simulink model "automotive_console_test"  (R2020b)
settings: Solver=VariableStepAuto  StartTime=0.0  StopTime=10.0  RelTol=1e-3
undefined symbols (not defined in the file): sigbuilder_block
settings Model: Creator=Milind  LastModifiedBy=Milind

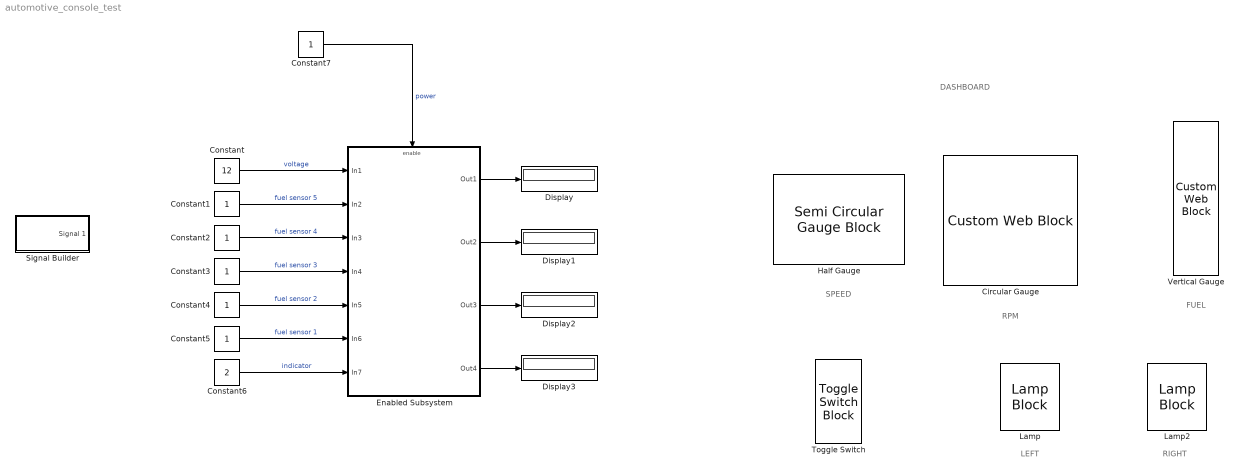
== system automotive_console_test ==
  note: LEFT
  note: SPEED
  note: DASHBOARD
  note: RIGHT
  note: RPM
  note: FUEL
  Circular Gauge : CustomWebBlock  LabelPosition=Hide  ShowInitialText=on  Configuration="{\"components\":[{\"name\":\"CircularScaleComponent\",\"settings\":{\"bounds\":{\"max\":10,\"min\":0,\"tickInterval\":\"auto\"},\"direction\":\"cw\",\"flipLimits\":0,\"innerRadius\":0.75,\"internalTickHeightScaleFactor\":1,\"labelColor\":[255,252,199],\"labelFont\":{\"font\":\"Arial\",\"fontSize\":12},\"labelTransparency\":1,\"minorTickHeightScaleFactor\":0.2,\"needleImage\":{\"size\":[1890,567],\"src\":\"data:image\\/svg+xml;base64,PD94bWwgdmVyc2lvbj0iMS4wIiBlbmNvZGluZz0iVVRGLTgiIHN0YW5kYWxvbmU9Im5vIj8+CjxzdmcKICAgeG1sbnM6ZGM9Imh0dHA6Ly9wdXJsLm9yZy9kYy9lbGVtZW50cy8xLjEvIgogICB4bWxuczpjYz0iaHR0cDovL2NyZWF0aXZlY29tbW9ucy5vcmcvbnMjIgogICB4bWxuczpyZGY9Imh0dHA6Ly93d3cudzMub3JnLzE5OTkvMDIvMjItcmRmLXN5bnRheC1ucyMiCiAgIHhtbG5zOnN2Zz0iaHR0cDovL3d3dy53My5vcmcvMjAwMC9zdmciCiAgIHhtbG5zPSJodHRwOi8vd3d3LnczLm9yZy8yMDAwL3N2ZyIKICAgeG1sbnM6 ...(+4096 chars)\"},\"needleOffset\":[0.1610917094974375,0],\"needleOrientation\":-45,\"needleRotation\":180.59702388394928,\"needleSize\":{\"height\":0.13032601008944536,\"width\":0.416859542883425},\"outerRadius\":0.9,\"position\":[0.06486742424242424,0.05627705627705628,0.8917748917748918,0.8787878787878788],\"scaleAngle\":270,\"scaleAngleOffset\":135,\"scaleColors\":[],\"scaleColorsSize\":0.2,\"scalePosition\":[0,0,1,1],\"showLabels\":1,\"showMinorTicks\":1,\"showSpanLine\":1,\"showTicks\":1,\"tickColor\":[255,255,200],\"tickTransparency\":1,\"valueBarColor\":[0,114,189],\"valueBarPosition\":[0,0,1,1],\"valueBarSize\":0.2,\"valueBarTransparency\":1}},{\"name\":\"BackgroundImageComponent\",\"settings\":{\"image\":{\"size\":[500,500],\"src\":\"data:image\\/svg+xml;base64,PD94bWwgdmVyc2lvbj0iMS4wIiBlbmNvZGluZz0iVVRGLTgiIHN0YW5kYWxvbmU9Im5vIj8+CjxzdmcKICAgeG1sbnM6ZGM9Imh0dHA6Ly9wdXJsLm9yZy9kYy9lbGVtZW50cy8xLjEvIgogICB4bWxuczpjYz0iaHR0cDovL2NyZWF0aXZlY29tbW9ucy5vcmcvbnMjIgogICB4bWxuczpyZGY9Imh0dHA6Ly93d3cudzMub3JnLzE5OTkvMDIvMjItcmRmLXN5bnRheC1ucyMiCiAgIHhtbG5zOnN2Zz0iaHR0cDovL3d3dy53My5vcmcvMjAwMC9zdmciCiAgIHhtbG5zPSJodHRwOi8vd3d3LnczLm9yZy8yMDAwL3N2ZyIKICAgeG1sbnM6 ...(+9964 chars)\"},\"position\":[0,0,1,1],\"scaleMode\":\"0\"}},{\"name\":\"ForegroundImageComponent\",\"settings\":{\"image\":{\"size\":[0,0],\"src\":\"default\",\"srcOrientation\":[]},\"isForeground\":1,\"position\":[0,0,1,1],\"scaleMode\":\"0\"}}],\"settings\":{\"BindingType\":\"signal\",\"aspectRatio\":1.032258064516129,\"direction\":\"cw\",\"fixedAspectRatio\":\"on\",\"flipLimits\":0,\"orientation\":\"horizontal\"},\"type\":\"CircularGauge\"}"
  Constant : Constant  Value=12
  Constant{1..5,7} (6 alike) : Constant
  Constant6 : Constant  Value=2
  Display{,1..3} (4 alike) : Display
  Enabled Subsystem : Subsystem  TreatAsAtomicUnit=on
  Half Gauge : SemiCircularGaugeBlock
  Lamp : LampBlock
  Lamp2 : LampBlock
  Signal Builder : Subsystem  Tag=STV Subsys  LoadFcn=sigbuilder_block('load');  StartFcn=sigbuilder_block('start');  StopFcn=sigbuilder_block('stop');  ClipboardFcn=sigbuilder_block('clipboard');  mask(Sigbuilder block){tuvar=[0:10]}
      mask help: Simulink:masks:SigbuilderBlock_MD
      mask init:
      | if ~strcmp(get_param(bdroot(gcbh),'SimulationStatus'),'stopped') tuvar = sigbuilder_block('maskInit'); end
      settings: CopyFcn=sigbuilder_block('copy');  DeleteFcn=sigbuilder_block('delete');  ModelCloseFcn=sigbuilder_block('modelClose');  PreSaveFcn=sigbuilder_block('preSave');  PauseFcn=sigbuilder_block('pause');  ContinueFcn=sigbuilder_block('continue');  NameChangeFcn=sigbuilder_block('namechange');  OpenFcn=sigbuilder_block('open',[437.6 153 550.4 359.25 ]);  CloseFcn=sigbuilder_block('close');
      mask Display: plot(0, 0, 100, 100,[2, 2, 32, 32, 2], [68, 8, 8, 68, 68],[32, 2], [38, 38], [32, 19, 2],[53, 60, 44], [32, 17, 17, 2],[16, 16, 31, 31]);txt = getActiveGroup(gcbh);text(2, 100, txt,'verticalAlignment', 'top');
  Toggle Switch : ToggleSwitchBlock
      settings: Values={{'Off', 'On'}, [0 1]}
  Vertical Gauge : CustomWebBlock  ShowInitialText=on  Configuration="{\"components\":[{\"name\":\"LinearScaleComponent\",\"settings\":{\"bounds\":{\"max\":5,\"min\":0,\"tickInterval\":\"auto\"},\"internalTickHeightScaleFactor\":0.5,\"labelColor\":[250,245,199],\"labelFont\":{\"font\":\"Arial\",\"fontSize\":12},\"labelTransparency\":1,\"needleImage\":{\"size\":[21,75],\"src\":\"data:image\\/svg+xml;base64,PHN2ZyB4bWxucz0iaHR0cDovL3d3dy53My5vcmcvMjAwMC9zdmciIHhtbG5zOnhsaW5rPSJodHRwOi8vd3d3LnczLm9yZy8xOTk5L3hsaW5rIiB2aWV3Qm94PSIwIDAgMjEgNzUiPjxkZWZzPjxzdHlsZT4uY2xzLTF7ZmlsbDpub25lO30uY2xzLTJ7aXNvbGF0aW9uOmlzb2xhdGU7fS5jbHMtM3tjbGlwLXBhdGg6dXJsKCNjbGlwLXBhdGgpO30uY2xzLTR7b3BhY2l0eTowLjM7bWl4LWJsZW5kLW1vZGU6bXVsdGlwbHk7fS5jbHMtNXtmaWxsOiNlYjI2Mjk7fTwvc3R5bGU+PGNsaXBQYXRoIGlkPSJjbGlwLXBhdGgiIHRyYW5zZm9y ...(+1928 chars)\",\"srcOrientation\":\"horizontal\"},\"needleOffset\":[-0.01094391244870041,0],\"needleSize\":{\"height\":0.11960078534031414,\"width\":0.7589285714285714},\"position\":[0.015887605042016806,0.06986607142857143,0.8,0.9641544117647058],\"scaleColors\":[],\"scaleColorsSize\":0.2,\"showLabels\":1,\"showMinorTicks\":0,\"showSpanLine\":1,\"showTicks\":1,\"tickColor\":[250,245,200],\"tickTransparency\":1,\"valueBarColor\":[23,89,176],\"valueBarOffset\":0,\"valueBarSize\":0.23,\"valueBarTransparency\":1}},{\"name\":\"BackgroundImageComponent\",\"settings\":{\"image\":{\"size\":[101,380],\"src\":\"data:image\\/svg+xml;base64,PHN2ZyB4bWxucz0iaHR0cDovL3d3dy53My5vcmcvMjAwMC9zdmciIHZpZXdCb3g9IjAgMCAxMDEgMzgwIj48ZGVmcz48c3R5bGU+LmNscy0xe2ZpbGw6IzAwMmI0Mjt9LmNscy0ye2ZpbGw6IzQyNzA4Mjt9LmNscy0ze2ZpbGw6IzdjYTBiMjt9PC9zdHlsZT48L2RlZnM+PHRpdGxlPnZlcnRpY2FsX2dhdWdlX2JhY2tncm91bmRfMTwvdGl0bGU+PGcgaWQ9IkxheWVyXzIiIGRhdGEtbmFtZT0iTGF5ZXIgMiI+PGcgaWQ9IkxheWVyXzEtMiIgZGF0YS1uYW1lPSJMYXllciAxIj48cmVjdCBjbGFzcz0iY2xzLTEiIHg9IjExIiB5PSIxMSIgd2lkdGg9Ijc5IiBoZWlnaHQ9IjM1OCIvPjxwYXRoIGNsYXNzPSJjbHMtMiIgZD0iTTkzLDhIOFYzNzJIOTNaTTExLDM2OVYxMUg5MFYzNjlaIi8+PHBhdGggY2xhc3M9ImNscy0zIiBkPSJNMTAxLDBIMFYzODBIMTAxWk04LDM3MlY4SDkzVjM3MloiLz48L2c+PC9nPjwvc3ZnPg==\",\"srcOrientation\":\"vertical\"},\"position\":[0,0,1,1],\"scaleMode\":\"0\"}},{\"name\":\"ForegroundImageComponent\",\"settings\":{\"image\":{\"size\":[0,0],\"src\":\"default\",\"srcOrientation\":[]},\"isForeground\":1,\"position\":[0,0,1,1],\"scaleMode\":\"0\"}}],\"settings\":{\"BindingType\":\"signal\",\"aspectRatio\":0.2647058823529412,\"fixedAspectRatio\":\"on\",\"orientation\":\"vertical\"},\"type\":\"LinearGauge\"}"
  wires:
  Enabled Subsystem/2(Out2) -> Display1/1
  Enabled Subsystem/3(Out3) -> Display2/1
  Constant2/1 -> Enabled Subsystem/3(In3)  "fuel sensor 4"
  Enabled Subsystem/1(Out1) -> Display/1
  Enabled Subsystem/4(Out4) -> Display3/1
  Constant7/1 -> Enabled Subsystem/Enable  "power"
  Constant5/1 -> Enabled Subsystem/6(In6)  "fuel sensor 1"
  Constant3/1 -> Enabled Subsystem/4(In4)  "fuel sensor 3"
  Constant6/1 -> Enabled Subsystem/7(In7)  "indicator"
  Constant4/1 -> Enabled Subsystem/5(In5)  "fuel sensor 2"
  Constant/1 -> Enabled Subsystem/1(In1)  "voltage"
  Constant1/1 -> Enabled Subsystem/2(In2)  "fuel sensor 5"

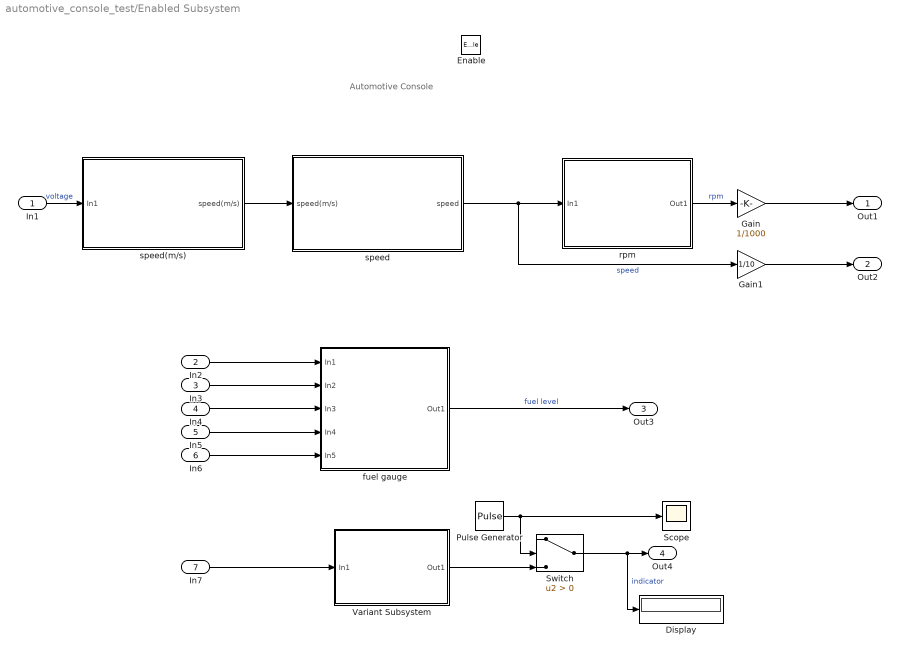
== system automotive_console_test/Enabled Subsystem ==
  note: Automotive Console
  In1 : Inport
  In2 : Inport  Port=2
  In3 : Inport  Port=3
  In4 : Inport  Port=4
  In5 : Inport  Port=5
  In6 : Inport  Port=6
  In7 : Inport  Port=7
  Enable : EnablePort
  Display : Display
  Gain : Gain  Gain=1/1000
  Gain1 : Gain  Gain=1/10
  Pulse Generator : DiscretePulseGenerator  PulseType=Time based  PulseWidth=50
  Scope : Scope
  Switch : Switch  Criteria=u2 > Threshold
  Variant Subsystem : Subsystem  Variant=on
  fuel gauge : Subsystem
  rpm : Subsystem  Variant=on
  speed : Subsystem  Variant=on  AllowZeroVariantControls=on
  speed(m/s) : Subsystem
  Out1 : Outport
  Out2 : Outport  Port=2
  Out3 : Outport  Port=3
  Out4 : Outport  Port=4
  wires:
  fuel gauge/1(Out1) -> Out3/1  "fuel level"
  Variant Subsystem/1(Out1) -> Switch/3
  speed/1(speed) -> Gain1/1, rpm/1(In1)  "speed"
  In2/1 -> fuel gauge/1(In1)
  In3/1 -> fuel gauge/2(In2)
  In4/1 -> fuel gauge/3(In3)
  rpm/1(Out1) -> Gain/1  "rpm"
  Pulse Generator/1 -> Scope/1, Switch/2
  In5/1 -> fuel gauge/4(In4)
  In7/1 -> Variant Subsystem/1(In1)
  In1/1 -> speed(m/s)/1(In1)  "voltage"
  In6/1 -> fuel gauge/5(In5)
  speed(m/s)/1(speed(m/s)) -> speed/1(speed(m/s))
  Switch/1 -> Display/1, Out4/1  "indicator"
  Gain/1 -> Out1/1
  Gain1/1 -> Out2/1

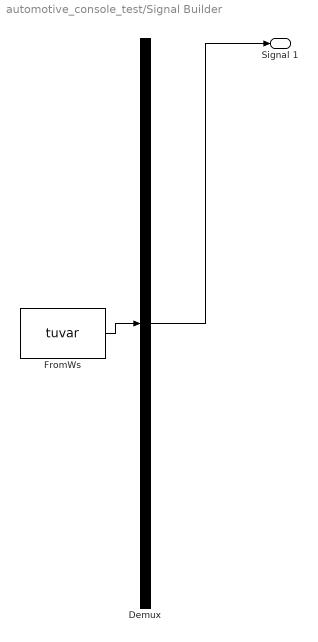
== system automotive_console_test/Signal Builder ==
  Demux : Demux  Tag=STV Demux  Outputs=1
      settings: DisplayOption=none
  FromWs : FromWorkspace  Tag=STV FromWs  VariableName=tuvar
      SigBuilderData=|
      | common.afterFinalStr = 'Extrapolate'
      | common.sampleTime = 0
      | dataSet.timeRange = [0 10]
      | dataSet.name = 'Group 1'
      | sbobj.Groups.Name = 'Group 1'
      | sbobj.Groups.Signals.Name = 'Signal 1'
      | sbobj.Groups.Signals.XData = [0 4 4 6 6 10]
      | sbobj.Groups.Signals.YData = [0 0 1 1 0 0]
  Signal 1 : Outport  Tag=STV Outport
  wires:
  Demux/1 -> Signal 1/1
  FromWs/1 -> Demux/1

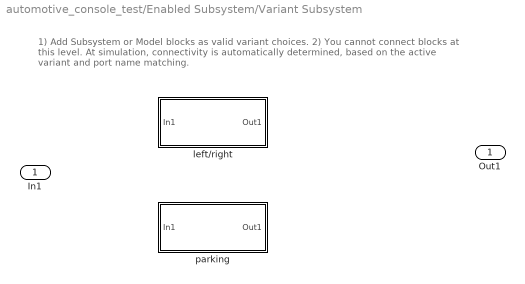
== system automotive_console_test/Enabled Subsystem/Variant Subsystem ==
  note: 1) Add Subsystem or Model blocks as valid variant choices.
      | 2) You cannot connect blocks at this level. At simulation, connectivity is automatically
      | determined, based on the active variant and port name matching.
  In1 : Inport
  left/right : Subsystem  VariantControl=ind==0
  parking : Subsystem  VariantControl=ind==1
  Out1 : Outport

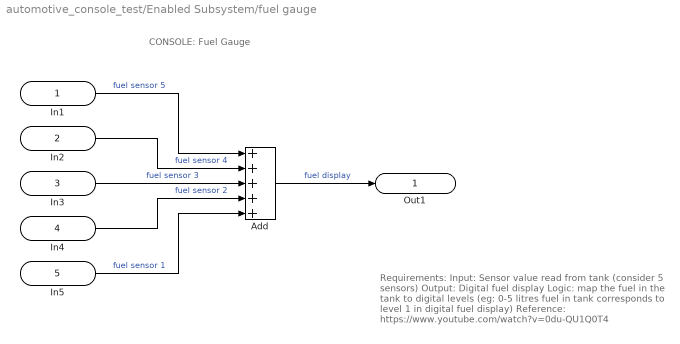
== system automotive_console_test/Enabled Subsystem/fuel gauge ==
  note: CONSOLE: Fuel Gauge
  note: Requirements:
      | Input: Sensor value read from tank (consider 5 sensors)
      | Output: Digital fuel display
      | Logic: map the fuel in the tank to digital levels (eg: 0-5 litres fuel in tank corresponds to level 1 in digital fuel display) Reference: https://www.youtube.com/watch?v=0du-QU1Q0T4
  In1 : Inport
  In2 : Inport  Port=2
  In3 : Inport  Port=3
  In4 : Inport  Port=4
  In5 : Inport  Port=5
  Add : Sum  Inputs=+++++
  Out1 : Outport
  wires:
  Add/1 -> Out1/1  "fuel display"
  In1/1 -> Add/1  "fuel sensor 5"
  In2/1 -> Add/2  "fuel sensor 4"
  In3/1 -> Add/3  "fuel sensor 3"
  In4/1 -> Add/4  "fuel sensor 2"
  In5/1 -> Add/5  "fuel sensor 1"

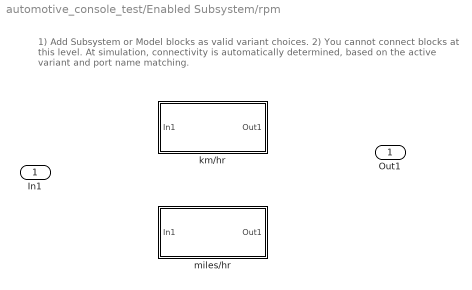
== system automotive_console_test/Enabled Subsystem/rpm ==
  note: 1) Add Subsystem or Model blocks as valid variant choices.
      | 2) You cannot connect blocks at this level. At simulation, connectivity is automatically
      | determined, based on the active variant and port name matching.
  In1 : Inport
  km/hr : Subsystem  VariantControl=control==0
  miles/hr : Subsystem  VariantControl=control==1
  Out1 : Outport

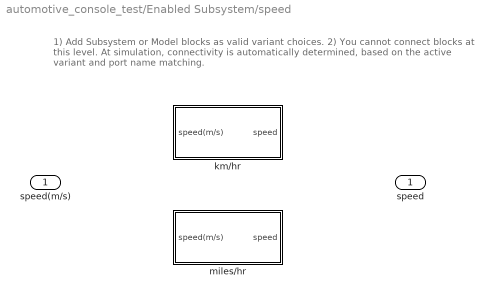
== system automotive_console_test/Enabled Subsystem/speed ==
  note: 1) Add Subsystem or Model blocks as valid variant choices.
      | 2) You cannot connect blocks at this level. At simulation, connectivity is automatically
      | determined, based on the active variant and port name matching.
  speed(m/s) : Inport
  km/hr : Subsystem  VariantControl=control==0
  miles/hr : Subsystem  VariantControl=control==1
  speed : Outport

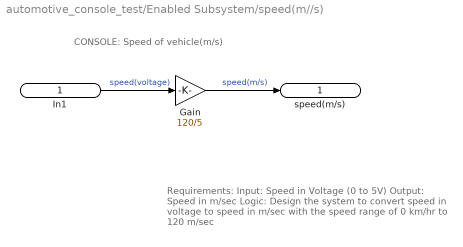
== system automotive_console_test/Enabled Subsystem/speed(m//s) ==
  note: CONSOLE: Speed of vehicle(m/s)
  note: Requirements:
      | Input: Speed in Voltage (0 to 5V)
      | Output: Speed in m/sec
      | Logic: Design the system to convert speed in voltage to
      | speed in m/sec with the speed range of 0 km/hr to 120 m/sec
  In1 : Inport
  Gain : Gain  Gain=120/5
  speed(m/s) : Outport
  wires:
  In1/1 -> Gain/1  "speed(voltage)"
  Gain/1 -> speed(m/s)/1  "speed(m/s)"

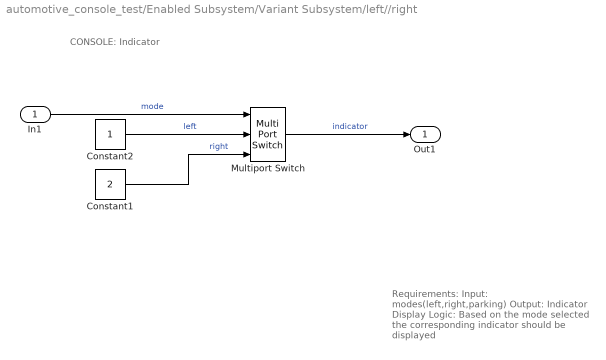
== system automotive_console_test/Enabled Subsystem/Variant Subsystem/left//right ==
  note: Requirements:
      | Input: modes(left,right,parking)
      | Output: Indicator Display
      | Logic: Based on the mode selected the corresponding indicator should be displayed
  note: CONSOLE: Indicator
  In1 : Inport
  Constant1 : Constant  Value=2
  Constant2 : Constant
  Multiport Switch : MultiPortSwitch  Inputs=2
  Out1 : Outport
  wires:
  In1/1 -> Multiport Switch/1  "mode"
  Constant1/1 -> Multiport Switch/3  "right"
  Constant2/1 -> Multiport Switch/2  "left"
  Multiport Switch/1 -> Out1/1  "indicator"

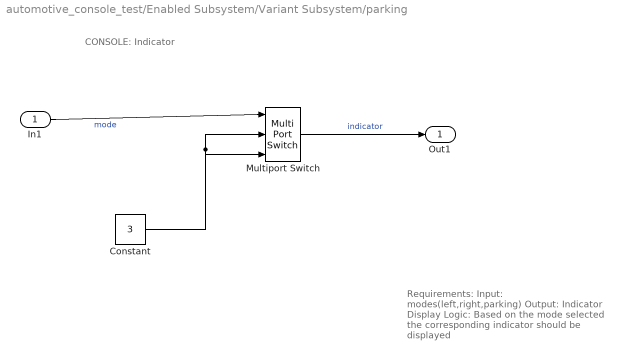
== system automotive_console_test/Enabled Subsystem/Variant Subsystem/parking ==
  note: Requirements:
      | Input: modes(left,right,parking)
      | Output: Indicator Display
      | Logic: Based on the mode selected the corresponding indicator should be displayed
  note: CONSOLE: Indicator
  In1 : Inport
  Constant : Constant  Value=3
  Multiport Switch : MultiPortSwitch  Inputs=2
  Out1 : Outport
  wires:
  Constant/1 -> Multiport Switch/3, Multiport Switch/2
  In1/1 -> Multiport Switch/1  "mode"
  Multiport Switch/1 -> Out1/1  "indicator"

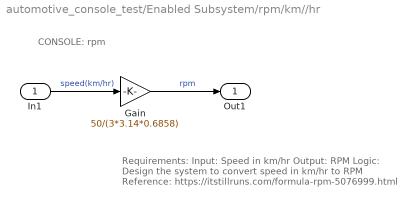
== system automotive_console_test/Enabled Subsystem/rpm/km//hr ==
  note: Requirements:
      | Input: Speed in km/hr
      | Output: RPM
      | Logic: Design the system to convert speed in km/hr to RPM Reference: https://itstillruns.com/formula-rpm-5076999.html
  note: CONSOLE: rpm
  In1 : Inport
  Gain : Gain  Gain=50/(3*3.14*0.6858)
  Out1 : Outport
  wires:
  Gain/1 -> Out1/1  "rpm"
  In1/1 -> Gain/1  "speed(km/hr)"

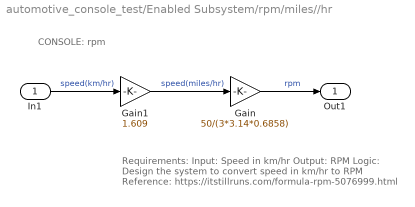
== system automotive_console_test/Enabled Subsystem/rpm/miles//hr ==
  note: Requirements:
      | Input: Speed in km/hr
      | Output: RPM
      | Logic: Design the system to convert speed in km/hr to RPM Reference: https://itstillruns.com/formula-rpm-5076999.html
  note: CONSOLE: rpm
  In1 : Inport
  Gain : Gain  Gain=50/(3*3.14*0.6858)
  Gain1 : Gain  Gain=1.609
  Out1 : Outport
  wires:
  Gain/1 -> Out1/1  "rpm"
  In1/1 -> Gain1/1  "speed(km/hr)"
  Gain1/1 -> Gain/1  "speed(miles/hr)"

== system automotive_console_test/Enabled Subsystem/speed/km//hr ==
  note: Requirements:
      | Input: Speed in m/sec
      | Output: Speed in km/hr
      | Logic: Design the system to convert speed from m/sec to km/hr
  note: CONSOLE: Speed of vehicle(km/hr)
  speed(m/s) : Inport
  Gain : Gain  Gain=3.6
  speed : Outport
  wires:
  Gain/1 -> speed/1
  speed(m/s)/1 -> Gain/1

== system automotive_console_test/Enabled Subsystem/speed/miles//hr ==
  note: Requirements:
      | Input: Speed in m/sec
      | Output: Speed in miles/hr
      | Logic: Design the system to convert speed from m/sec to miles/hr
  note: CONSOLE: Speed of vehicle(miles/hr)
  speed(m/s) : Inport
  Gain1 : Gain  Gain=2.237
  speed : Outport
  wires:
  Gain1/1 -> speed/1
  speed(m/s)/1 -> Gain1/1
